simulink model "fun_call_outputEvent_mulBrodcast_eg"  (R2018a)
settings: Solver=VariableStepAuto  StartTime=0.0  StopTime=10.0  RelTol=1e-3
settings Model: Creator=86188  LastModifiedBy=86188

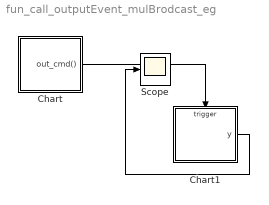
== system fun_call_outputEvent_mulBrodcast_eg ==
  Chart : Stateflow chart  TreatAsAtomicUnit=on
  Chart1 : Stateflow chart  TreatAsAtomicUnit=on
  Scope : Scope
  wires:
  Chart/1(out_cmd()) -> Chart1/Trigger
  Chart1/1(y) -> Scope/1

== stateflow chart fun_call_outputEvent_mulBrodcast_eg/Chart1 ==
  settings: executeAtInitialization=1
  (default) -> (junction 1) : {y = y + 1;}
  data: y output =0
  events: out_cmd input FUNCTION_CALL_EVENT

== stateflow chart fun_call_outputEvent_mulBrodcast_eg/Chart ==
  state ENTRY
  state A
    en:
    send(out_cmd);
    send(out_cmd);
    send(out_cmd);
    send(out_cmd);
  state B
  (default) -> ENTRY
  A -> B
  ENTRY -> A
  events: out_cmd output FUNCTION_CALL_EVENT
